simulink model "main"  (R2025b)
settings: Solver=ode1  StartTime=0.0  StopTime=config.sim.var.sim_time  FixedStep=config.sim.var.time_step  RelTol=1e-3
PreLoadFcn:
  | addpath(fullfile(pwd,'images'));
InitFcn:
  | run(fullfile(fileparts(get_param(bdroot,'FileName')),'initializer.mlx'))
StopFcn:
  | run(fullfile(fileparts(get_param(bdroot,'FileName')),'plot/plotting_results.m'))
undefined symbols (not defined in the file): config
libraries: simulink x8, sharedTrackingLibrary x2
(part 1 of 2)
settings Model: Creator=Diogo Lima  LastModifiedBy=Diogo Lima
settings DataIOCC: ExternalInput=config

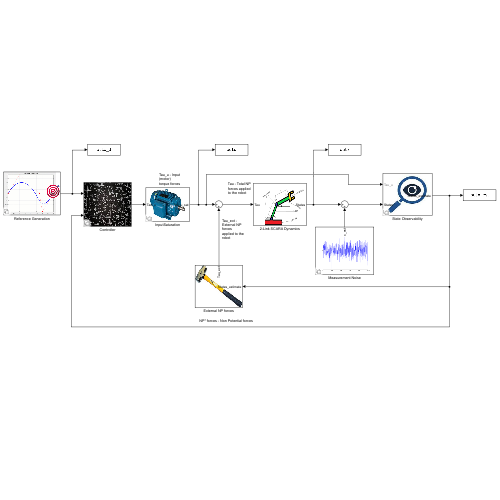
[thumbnail: Simulink's stored preview of the top-level diagram]
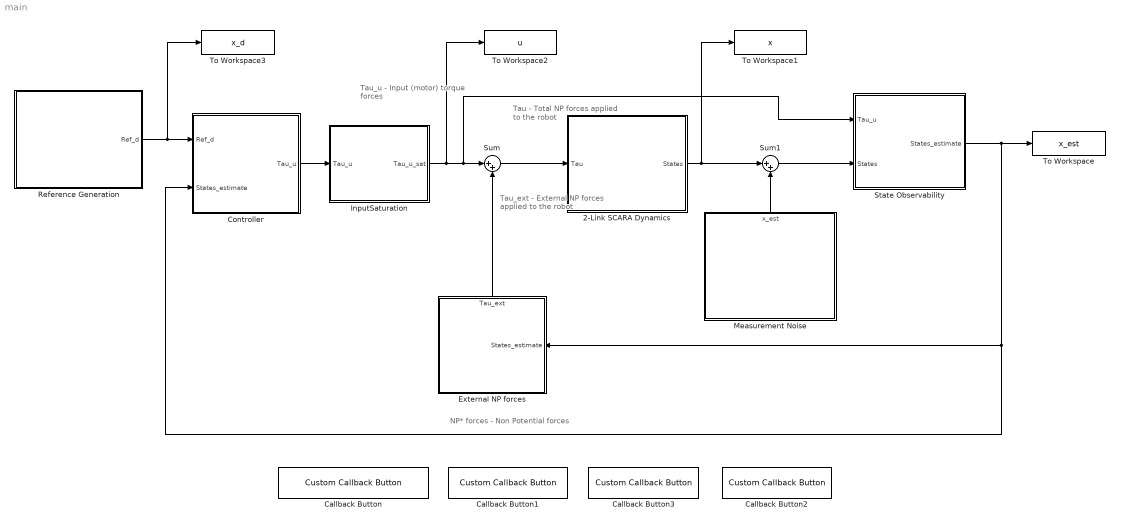
== system main ==
  note: NP* forces - Non Potential forces
  note: Tau - Total NP forces applied to the robot
  note: Tau_u - Input (motor) torque forces
  note: Tau_ext - External NP forces applied to the robot
  2-Link SCARA Dynamics : Subsystem
      mask Display: image('2_Link_Rob_Arm.png');
  Callback Button : CustomCallbackButton  Configuration="{\"components\":[{\"name\":\"BackgroundImageComponent\",\"settings\":{\"image\":{\"size\":[0,0],\"src\":\"default\",\"srcOrientation\":\"Right\"},\"position\":[0,0,1,1]}},{\"name\":\"ButtonStateComponent\",\"settings\":{\"buttonType\":\"momentary\",\"clickFcn\":\"PlotStatesEstDes(plotData);\",\"onValue\":1,\"position\":[0,0,1,1],\"pressDelay\":\"500\",\"pressFcn\":\"\",\"repeatInterval\":\"0\",\"states\":[{\"horizontalAlignment\":\"center\",\"image\":{\"position\":[0,0,1,1],\"size\":[1,1],\"src\":\"default\",\"srcOrientation\":\"Right\"},\"label\":{\"color\":[0.01176470588,0.01176470588,0.01176470588,1],\"icon\":{\"size\":[0,0],\"src\":\"default\",\"srcOrientation\":\"Right\"},\"iconOffset\":0,\"iconPlacement\":\"left\",\"opacity\":1,\"show\":true,\"text\":{\"content\":\"Plot x, x_est and x_d\",\"font\":\"Helvetica\"}},\"labelOffset\":[0,0],\"verticalAlignment\":\"middle\"},{\"horizontalAlignment\":\"center\",\"image\":{\"position\":[0,0,1,1],\"size\":[1,1],\"src\":\"default\",\"srcOrientation\":\"Right\"},\"label\":{\"color\":[0.01176470588,0.01176470588,0.01176470588,1],\"icon\":{\"size\":[0,0],\"src\":\"default\",\"srcOrientation\":\"Right\"},\"iconOffset\":0,\"iconPlacement\":\"left\",\"opacity\":1,\"show\":true,\"text\":{\"content\":\"Plot x, x_est and x_d\",\"font\":\"Helvetica\"}},\"labelOffset\":[0,0],\"verticalAlignment\":\"middle\"},{\"horizontalAlignment\":\"center\",\"image\":{\"position\":[0,0,1,1],\"size\":[1,1],\"src\":\"default\",\"srcOrientation\":\"Right\"},\"label\":{\"color\":[0.01176470588,0.01176470588,0.01176470588,1],\"icon\":{\"size\":[0,0],\"src\":\"default\",\"srcOrientation\":\"Right\"},\"iconOffset\":0,\"iconPlacement\":\"left\",\"opacity\":1,\"show\":true,\"text\":{\"content\":\"Plot x, x_est and x_d\",\"font\":\"Helvetica\"}},\"labelOffset\":[0,0],\"verticalAlignment\":\"middle\"},{\"horizontalAlignment\":\"center\",\"image\":{\"position\":[0,0,1,1],\"size\":[1,1],\"src\":\"default\",\"srcOrientation\":\"Right\"},\"label\":{\"color\":[0.01176470588,0.01176470588,0.01176470588,1],\"icon\":{\"size\":[0,0],\"src\":\"default\",\"srcOrientation\":\"Right\"},\"iconOffset\":0,\"iconPlacement\":\"left\",\"opacity\":1,\"show\":true,\"text\":{\"content\":\"Plot x, x_est and x_d\",\"font\":\"Helvetica\"}},\"labelOffset\":[0,0],\"verticalAlignment\":\"middle\"}]}},{\"name\":\"ForegroundImageComponent\",\"settings\":{\"image\":{\"size\":[0,0],\"src\":\"default\",\"srcOrientation\":\"Right\"},\"isForeground\":1,\"position\":[0,0,1,1]}}],\"derived\":{\"blockParameters\":{\"AutoActivate\":true,\"ButtonText\":\"Plot x, x_est and x_d\",\"ButtonType\":\"Momentary\",\"ClickFcn\":\"PlotStatesEstDes(plotData);\",\"OnValue\":1,\"PressDelay\":\"500\",\"PressFcn\":\"\",\"RepeatInterval\":\"0\",\"fixedAspectRatio\":\"off\"}},\"settings\":{\"BindingType\":\"standalone\",\"autoActivate\":true,\"backgroundColor\":[244,244,244,1],\"backgroundOffset\":0.2,\"backgroundOpacity\":1,\"fixedAspectRatio\":\"off\",\"foregroundColor\":[0.01176470588,0.01176470588,0.01176470588,1],\"migratedFromLegacy\":true,\"useBackgroundColor\":true,\"variant\":\"callback\",\"version\":\"R2025a\"},\"type\":\"Button\"}"  CustomBackgroundColor="{\"color\":[0.9568627451,0.9568627451,0.9568627451],\"show\":true}"
  Callback Button1 : CustomCallbackButton  Configuration="{\"components\":[{\"name\":\"BackgroundImageComponent\",\"settings\":{\"image\":{\"size\":[0,0],\"src\":\"default\",\"srcOrientation\":\"Right\"},\"position\":[0,0,1,1]}},{\"name\":\"ButtonStateComponent\",\"settings\":{\"buttonType\":\"momentary\",\"clickFcn\":\"PlotError(plotData, config);\",\"onValue\":1,\"position\":[0,0,1,1],\"pressDelay\":\"500\",\"pressFcn\":\"\",\"repeatInterval\":\"0\",\"states\":[{\"horizontalAlignment\":\"center\",\"image\":{\"position\":[0,0,1,1],\"size\":[1,1],\"src\":\"default\",\"srcOrientation\":\"Right\"},\"label\":{\"color\":[0.01176470588,0.01176470588,0.01176470588,1],\"icon\":{\"size\":[0,0],\"src\":\"default\",\"srcOrientation\":\"Right\"},\"iconOffset\":0,\"iconPlacement\":\"left\",\"opacity\":1,\"show\":true,\"text\":{\"content\":\"Plot Errors\",\"font\":\"Helvetica\"}},\"labelOffset\":[0,0],\"verticalAlignment\":\"middle\"},{\"horizontalAlignment\":\"center\",\"image\":{\"position\":[0,0,1,1],\"size\":[1,1],\"src\":\"default\",\"srcOrientation\":\"Right\"},\"label\":{\"color\":[0.01176470588,0.01176470588,0.01176470588,1],\"icon\":{\"size\":[0,0],\"src\":\"default\",\"srcOrientation\":\"Right\"},\"iconOffset\":0,\"iconPlacement\":\"left\",\"opacity\":1,\"show\":true,\"text\":{\"content\":\"Plot Errors\",\"font\":\"Helvetica\"}},\"labelOffset\":[0,0],\"verticalAlignment\":\"middle\"},{\"horizontalAlignment\":\"center\",\"image\":{\"position\":[0,0,1,1],\"size\":[1,1],\"src\":\"default\",\"srcOrientation\":\"Right\"},\"label\":{\"color\":[0.01176470588,0.01176470588,0.01176470588,1],\"icon\":{\"size\":[0,0],\"src\":\"default\",\"srcOrientation\":\"Right\"},\"iconOffset\":0,\"iconPlacement\":\"left\",\"opacity\":1,\"show\":true,\"text\":{\"content\":\"Plot Errors\",\"font\":\"Helvetica\"}},\"labelOffset\":[0,0],\"verticalAlignment\":\"middle\"},{\"horizontalAlignment\":\"center\",\"image\":{\"position\":[0,0,1,1],\"size\":[1,1],\"src\":\"default\",\"srcOrientation\":\"Right\"},\"label\":{\"color\":[0.01176470588,0.01176470588,0.01176470588,1],\"icon\":{\"size\":[0,0],\"src\":\"default\",\"srcOrientation\":\"Right\"},\"iconOffset\":0,\"iconPlacement\":\"left\",\"opacity\":1,\"show\":true,\"text\":{\"content\":\"Plot Errors\",\"font\":\"Helvetica\"}},\"labelOffset\":[0,0],\"verticalAlignment\":\"middle\"}]}},{\"name\":\"ForegroundImageComponent\",\"settings\":{\"image\":{\"size\":[0,0],\"src\":\"default\",\"srcOrientation\":\"Right\"},\"isForeground\":1,\"position\":[0,0,1,1]}}],\"derived\":{\"blockParameters\":{\"AutoActivate\":true,\"ButtonText\":\"Plot Errors\",\"ButtonType\":\"Momentary\",\"ClickFcn\":\"PlotError(plotData, config);\",\"OnValue\":1,\"PressDelay\":\"500\",\"PressFcn\":\"\",\"RepeatInterval\":\"0\",\"fixedAspectRatio\":\"off\"}},\"settings\":{\"BindingType\":\"standalone\",\"autoActivate\":true,\"backgroundColor\":[244,244,244,1],\"backgroundOffset\":0.2,\"backgroundOpacity\":1,\"fixedAspectRatio\":\"off\",\"foregroundColor\":[0.01176470588,0.01176470588,0.01176470588,1],\"migratedFromLegacy\":true,\"useBackgroundColor\":true,\"variant\":\"callback\",\"version\":\"R2025a\"},\"type\":\"Button\"}"  CustomBackgroundColor="{\"color\":[0.9568627451,0.9568627451,0.9568627451],\"show\":true}"
  Callback Button2 : CustomCallbackButton  Configuration="{\"components\":[{\"name\":\"BackgroundImageComponent\",\"settings\":{\"image\":{\"size\":[0,0],\"src\":\"default\",\"srcOrientation\":\"Right\"},\"position\":[0,0,1,1]}},{\"name\":\"ButtonStateComponent\",\"settings\":{\"buttonType\":\"momentary\",\"clickFcn\":\"Animate2LinkSCARA(plotData, config);\",\"onValue\":1,\"position\":[0,0,1,1],\"pressDelay\":\"500\",\"pressFcn\":\"\",\"repeatInterval\":\"0\",\"states\":[{\"horizontalAlignment\":\"center\",\"image\":{\"position\":[0,0,1,1],\"size\":[1,1],\"src\":\"default\",\"srcOrientation\":\"Right\"},\"label\":{\"color\":[0.01176470588,0.01176470588,0.01176470588,1],\"icon\":{\"size\":[0,0],\"src\":\"default\",\"srcOrientation\":\"Right\"},\"iconOffset\":0,\"iconPlacement\":\"left\",\"opacity\":1,\"show\":true,\"text\":{\"content\":\"Animation\",\"font\":\"Helvetica\"}},\"labelOffset\":[0,0],\"verticalAlignment\":\"middle\"},{\"horizontalAlignment\":\"center\",\"image\":{\"position\":[0,0,1,1],\"size\":[1,1],\"src\":\"default\",\"srcOrientation\":\"Right\"},\"label\":{\"color\":[0.01176470588,0.01176470588,0.01176470588,1],\"icon\":{\"size\":[0,0],\"src\":\"default\",\"srcOrientation\":\"Right\"},\"iconOffset\":0,\"iconPlacement\":\"left\",\"opacity\":1,\"show\":true,\"text\":{\"content\":\"Animation\",\"font\":\"Helvetica\"}},\"labelOffset\":[0,0],\"verticalAlignment\":\"middle\"},{\"horizontalAlignment\":\"center\",\"image\":{\"position\":[0,0,1,1],\"size\":[1,1],\"src\":\"default\",\"srcOrientation\":\"Right\"},\"label\":{\"color\":[0.01176470588,0.01176470588,0.01176470588,1],\"icon\":{\"size\":[0,0],\"src\":\"default\",\"srcOrientation\":\"Right\"},\"iconOffset\":0,\"iconPlacement\":\"left\",\"opacity\":1,\"show\":true,\"text\":{\"content\":\"Animation\",\"font\":\"Helvetica\"}},\"labelOffset\":[0,0],\"verticalAlignment\":\"middle\"},{\"horizontalAlignment\":\"center\",\"image\":{\"position\":[0,0,1,1],\"size\":[1,1],\"src\":\"default\",\"srcOrientation\":\"Right\"},\"label\":{\"color\":[0.01176470588,0.01176470588,0.01176470588,1],\"icon\":{\"size\":[0,0],\"src\":\"default\",\"srcOrientation\":\"Right\"},\"iconOffset\":0,\"iconPlacement\":\"left\",\"opacity\":1,\"show\":true,\"text\":{\"content\":\"Animation\",\"font\":\"Helvetica\"}},\"labelOffset\":[0,0],\"verticalAlignment\":\"middle\"}]}},{\"name\":\"ForegroundImageComponent\",\"settings\":{\"image\":{\"size\":[0,0],\"src\":\"default\",\"srcOrientation\":\"Right\"},\"isForeground\":1,\"position\":[0,0,1,1]}}],\"derived\":{\"blockParameters\":{\"AutoActivate\":true,\"ButtonText\":\"Animation\",\"ButtonType\":\"Momentary\",\"ClickFcn\":\"Animate2LinkSCARA(plotData, config);\",\"OnValue\":1,\"PressDelay\":\"500\",\"PressFcn\":\"\",\"RepeatInterval\":\"0\",\"fixedAspectRatio\":\"off\"}},\"settings\":{\"BindingType\":\"standalone\",\"autoActivate\":true,\"backgroundColor\":[244,244,244,1],\"backgroundOffset\":0.2,\"backgroundOpacity\":1,\"fixedAspectRatio\":\"off\",\"foregroundColor\":[0.01176470588,0.01176470588,0.01176470588,1],\"migratedFromLegacy\":true,\"useBackgroundColor\":true,\"variant\":\"callback\",\"version\":\"R2025a\"},\"type\":\"Button\"}"  CustomBackgroundColor="{\"color\":[0.9568627451,0.9568627451,0.9568627451],\"show\":true}"
  Callback Button3 : CustomCallbackButton  Configuration="{\"components\":[{\"name\":\"BackgroundImageComponent\",\"settings\":{\"image\":{\"size\":[0,0],\"src\":\"default\",\"srcOrientation\":\"Right\"},\"position\":[0,0,1,1]}},{\"name\":\"ButtonStateComponent\",\"settings\":{\"buttonType\":\"momentary\",\"clickFcn\":\"PlotInput(plotData, config);\",\"onValue\":1,\"position\":[0,0,1,1],\"pressDelay\":\"500\",\"pressFcn\":\"\",\"repeatInterval\":\"0\",\"states\":[{\"horizontalAlignment\":\"center\",\"image\":{\"position\":[0,0,1,1],\"size\":[1,1],\"src\":\"default\",\"srcOrientation\":\"Right\"},\"label\":{\"color\":[0.01176470588,0.01176470588,0.01176470588,1],\"icon\":{\"size\":[0,0],\"src\":\"default\",\"srcOrientation\":\"Right\"},\"iconOffset\":0,\"iconPlacement\":\"left\",\"opacity\":1,\"show\":true,\"text\":{\"content\":\"Input Torques\",\"font\":\"Helvetica\"}},\"labelOffset\":[0,0],\"verticalAlignment\":\"middle\"},{\"horizontalAlignment\":\"center\",\"image\":{\"position\":[0,0,1,1],\"size\":[1,1],\"src\":\"default\",\"srcOrientation\":\"Right\"},\"label\":{\"color\":[0.01176470588,0.01176470588,0.01176470588,1],\"icon\":{\"size\":[0,0],\"src\":\"default\",\"srcOrientation\":\"Right\"},\"iconOffset\":0,\"iconPlacement\":\"left\",\"opacity\":1,\"show\":true,\"text\":{\"content\":\"Input Torques\",\"font\":\"Helvetica\"}},\"labelOffset\":[0,0],\"verticalAlignment\":\"middle\"},{\"horizontalAlignment\":\"center\",\"image\":{\"position\":[0,0,1,1],\"size\":[1,1],\"src\":\"default\",\"srcOrientation\":\"Right\"},\"label\":{\"color\":[0.01176470588,0.01176470588,0.01176470588,1],\"icon\":{\"size\":[0,0],\"src\":\"default\",\"srcOrientation\":\"Right\"},\"iconOffset\":0,\"iconPlacement\":\"left\",\"opacity\":1,\"show\":true,\"text\":{\"content\":\"Input Torques\",\"font\":\"Helvetica\"}},\"labelOffset\":[0,0],\"verticalAlignment\":\"middle\"},{\"horizontalAlignment\":\"center\",\"image\":{\"position\":[0,0,1,1],\"size\":[1,1],\"src\":\"default\",\"srcOrientation\":\"Right\"},\"label\":{\"color\":[0.01176470588,0.01176470588,0.01176470588,1],\"icon\":{\"size\":[0,0],\"src\":\"default\",\"srcOrientation\":\"Right\"},\"iconOffset\":0,\"iconPlacement\":\"left\",\"opacity\":1,\"show\":true,\"text\":{\"content\":\"Input Torques\",\"font\":\"Helvetica\"}},\"labelOffset\":[0,0],\"verticalAlignment\":\"middle\"}]}},{\"name\":\"ForegroundImageComponent\",\"settings\":{\"image\":{\"size\":[0,0],\"src\":\"default\",\"srcOrientation\":\"Right\"},\"isForeground\":1,\"position\":[0,0,1,1]}}],\"derived\":{\"blockParameters\":{\"AutoActivate\":true,\"ButtonText\":\"Input Torques\",\"ButtonType\":\"Momentary\",\"ClickFcn\":\"PlotInput(plotData, config);\",\"OnValue\":1,\"PressDelay\":\"500\",\"PressFcn\":\"\",\"RepeatInterval\":\"0\",\"fixedAspectRatio\":\"off\"}},\"settings\":{\"BindingType\":\"standalone\",\"autoActivate\":true,\"backgroundColor\":[244,244,244,1],\"backgroundOffset\":0.2,\"backgroundOpacity\":1,\"fixedAspectRatio\":\"off\",\"foregroundColor\":[0.01176470588,0.01176470588,0.01176470588,1],\"migratedFromLegacy\":true,\"useBackgroundColor\":true,\"variant\":\"callback\",\"version\":\"R2025a\"},\"type\":\"Button\"}"  CustomBackgroundColor="{\"color\":[0.9568627451,0.9568627451,0.9568627451],\"show\":true}"
  Controller : Subsystem  Variant=on  VariantActivationTime=inherit from Simulink.VariantControl
      mask Display: image('math.jpeg');
  External NP forces : Subsystem
      settings: PortSchema="{\"entries\":[{\"content\":{\"sides\":[{\"content\":{},\"type\":\"ConnectorPlacement.EquallySpacedRectSide\",\"uuid\":\"ab8935ab-44b5-4f89-9c76-b9cab063ccb6\"},{\"content\":{\"connectorIds\":[\"In1\"],\"side\":\"RIGHT\"},\"type\":\"ConnectorPlacement.EquallySpacedRectSide\",\"uuid\":\"7b95b46e-af84-4841-baf6-a25fb8fbec5d\"},{\"content\":{\"connectorIds\":[\"Out1\"],\"side\":\"TOP\"},\"type\":\"ConnectorPlacement.EquallySpacedRectSide\",\"uuid\":\"f47b6b94-5272-4357-86f1-013d8bd46a68\"},{\"content\":{\"side\":\"BOTTOM\"},\"type\":\"ConnectorPlacement.EquallySpacedRectSide\",\"uuid\":\"e5ddd4d5-8d82-42eb-baf0-e1f1d67c3ee6\"}]},\"type\":\"ConnectorPlacement.EquallySpacedConnector\",\"uuid\":\"5043c8e4-624e-44a2-8db2-4a7bf2c36b25\"}],\"packageUris\":[\"http://schema.mathworks.com/mf0/Connector/R2020b\"],\"version\":\"1.0\"}"
      mask Display: image('hammer.jpeg');
  InputSaturation : Subsystem  Variant=on  VariantActivationTime=inherit from Simulink.VariantControl
      mask Display: image('eetric motor.jpeg');
  Measurement Noise : Subsystem  Variant=on  VariantActivationTime=inherit from Simulink.VariantControl
      settings: PortSchema="{\"entries\":[{\"content\":{\"sides\":[{\"content\":{},\"type\":\"ConnectorPlacement.EquallySpacedRectSide\",\"uuid\":\"d15af3bb-429c-4511-867e-2dbe032e8cba\"},{\"content\":{\"side\":\"RIGHT\"},\"type\":\"ConnectorPlacement.EquallySpacedRectSide\",\"uuid\":\"fe1fb238-6986-44a7-806c-ef391cb9083b\"},{\"content\":{\"connectorIds\":[\"Out1\"],\"side\":\"TOP\"},\"type\":\"ConnectorPlacement.EquallySpacedRectSide\",\"uuid\":\"1cb65108-e0a3-4597-9e58-247715da98e5\"}]},\"type\":\"ConnectorPlacement.EquallySpacedConnector\",\"uuid\":\"dec8af6e-1fcd-4cfd-bd39-6a634de96718\"}],\"packageUris\":[\"http://schema.mathworks.com/mf0/Connector/R2020b\"],\"version\":\"1.0\"}"
      mask Display: image('gussian_normal_noise.png');
  Reference Generation : Subsystem  Variant=on  VariantActivationTime=inherit from Simulink.VariantControl
      mask Display: image('Trajectory Target.png');
  State Observability : Subsystem  Variant=on  VariantActivationTime=inherit from Simulink.VariantControl
      mask Display: image('magnifying glass.jpeg');
  Sum : Sum  Inputs=|++
  Sum1 : Sum  Inputs=|++
  To Workspace : ToWorkspace  VariableName=x_est  SaveFormat=Structure With Time  SampleTime=-1
  To Workspace1 : ToWorkspace  VariableName=x  SaveFormat=Structure With Time  SampleTime=-1
  To Workspace2 : ToWorkspace  VariableName=u  SaveFormat=Structure With Time  SampleTime=-1
  To Workspace3 : ToWorkspace  VariableName=x_d  SaveFormat=Structure With Time  SampleTime=-1
  wires:
  2-Link SCARA Dynamics/1(States) -> Sum1/1, To Workspace1/1
  Sum/1 -> 2-Link SCARA Dynamics/1(Tau)
  External NP forces/1(Tau_ext) -> Sum/2
  Reference Generation/1(Ref_d) -> To Workspace3/1, Controller/1(Ref_d)
  Controller/1(Tau_u) -> InputSaturation/1(Tau_u)
  InputSaturation/1(Tau_u_sat) -> To Workspace2/1, State Observability/1(Tau_u), Sum/1
  State Observability/1(States_estimate) -> Controller/2(States_estimate), External NP forces/1(States_estimate), To Workspace/1
  Sum1/1 -> State Observability/2(States)
  Measurement Noise/1(x_est) -> Sum1/2

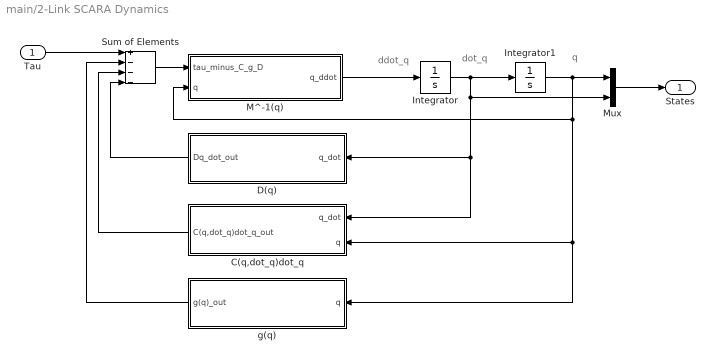
== system main/2-Link SCARA Dynamics ==
  note: dot_q
  note: q
  note: ddot_q
  Tau : Inport
  C(q,dot_q)dot_q : Subsystem
      settings: PortSchema="{\"entries\":[{\"content\":{\"sides\":[{\"content\":{\"connectorIds\":[\"Out1\"]},\"type\":\"ConnectorPlacement.EquallySpacedRectSide\",\"uuid\":\"e2ae5650-0784-458d-831f-709044d8d2e7\"},{\"content\":{\"connectorIds\":[\"In1\",\"In2\"],\"side\":\"RIGHT\"},\"type\":\"ConnectorPlacement.EquallySpacedRectSide\",\"uuid\":\"7d6ada7b-e0cb-4ab5-ae4d-653c8188ff73\"},{\"content\":{\"side\":\"TOP\"},\"type\":\"ConnectorPlacement.EquallySpacedRectSide\",\"uuid\":\"6bba282a-332d-41c7-9399-ff8c7d6086e4\"}]},\"type\":\"ConnectorPlacement.EquallySpacedConnector\",\"uuid\":\"9d2ac4ef-2b70-4a02-8c87-fdaaf2184e3a\"}],\"packageUris\":[\"http://schema.mathworks.com/mf0/Connector/R2020b\"],\"version\":\"1.0\"}"
  D(q) : Subsystem
      settings: PortSchema="{\"entries\":[{\"content\":{\"sides\":[{\"content\":{\"connectorIds\":[\"Out1\"]},\"type\":\"ConnectorPlacement.EquallySpacedRectSide\",\"uuid\":\"e2ae5650-0784-458d-831f-709044d8d2e7\"},{\"content\":{\"connectorIds\":[\"In1\"],\"side\":\"RIGHT\"},\"type\":\"ConnectorPlacement.EquallySpacedRectSide\",\"uuid\":\"7d6ada7b-e0cb-4ab5-ae4d-653c8188ff73\"},{\"content\":{\"side\":\"TOP\"},\"type\":\"ConnectorPlacement.EquallySpacedRectSide\",\"uuid\":\"6bba282a-332d-41c7-9399-ff8c7d6086e4\"}]},\"type\":\"ConnectorPlacement.EquallySpacedConnector\",\"uuid\":\"9d2ac4ef-2b70-4a02-8c87-fdaaf2184e3a\"}],\"packageUris\":[\"http://schema.mathworks.com/mf0/Connector/R2020b\"],\"version\":\"1.0\"}"
  Integrator : Integrator  InitialCondition=config.sim.var.init_cond.ang_vel
  Integrator1 : Integrator  InitialCondition=config.sim.var.init_cond.ang_pos
  M^-1(q) : Subsystem
  Mux : Mux  Inputs=2
  Sum of Elements : Sum  Inputs=+---
  g(q) : Subsystem
      settings: PortSchema="{\"entries\":[{\"content\":{\"sides\":[{\"content\":{\"connectorIds\":[\"Out1\"]},\"type\":\"ConnectorPlacement.EquallySpacedRectSide\",\"uuid\":\"e2ae5650-0784-458d-831f-709044d8d2e7\"},{\"content\":{\"connectorIds\":[\"In1\"],\"side\":\"RIGHT\"},\"type\":\"ConnectorPlacement.EquallySpacedRectSide\",\"uuid\":\"7d6ada7b-e0cb-4ab5-ae4d-653c8188ff73\"},{\"content\":{\"side\":\"TOP\"},\"type\":\"ConnectorPlacement.EquallySpacedRectSide\",\"uuid\":\"6bba282a-332d-41c7-9399-ff8c7d6086e4\"}]},\"type\":\"ConnectorPlacement.EquallySpacedConnector\",\"uuid\":\"9d2ac4ef-2b70-4a02-8c87-fdaaf2184e3a\"}],\"packageUris\":[\"http://schema.mathworks.com/mf0/Connector/R2020b\"],\"version\":\"1.0\"}"
  States : Outport
  wires:
  M^-1(q)/1(q_ddot) -> Integrator/1
  Integrator/1 -> C(q,dot_q)dot_q/1(q_dot), D(q)/1(q_dot), Mux/2, Integrator1/1
  Mux/1 -> States/1
  Integrator1/1 -> M^-1(q)/2(q), g(q)/1(q), C(q,dot_q)dot_q/2(q), Mux/1
  Sum of Elements/1 -> M^-1(q)/1(tau_minus_C_g_D)
  Tau/1 -> Sum of Elements/1
  D(q)/1(Dq_dot_out) -> Sum of Elements/4
  C(q,dot_q)dot_q/1(C(q,dot_q)dot_q_out) -> Sum of Elements/3
  g(q)/1(g(q)_out) -> Sum of Elements/2

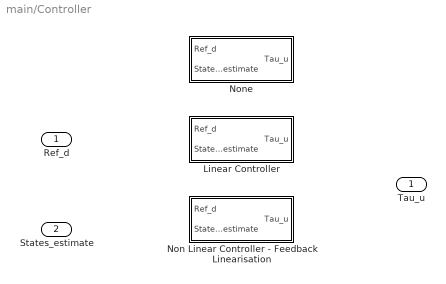
== system main/Controller ==
  Ref_d : Inport
  States_estimate : Inport  Port=2
  Linear Controller : Subsystem  VariantControl=ControllerSel == ControllerType.LinearSS
  Non Linear Controller - Feedback Linearisation : Subsystem  VariantControl=ControllerSel == ControllerType.NonLinearFL
  None : Subsystem  VariantControl=ControllerSel == ControllerType.None
  Tau_u : Outport

== system main/External NP forces ==
  States_estimate : Inport
  Add : Sum
  External Disturbance Forces / Model Uncertainties : Subsystem  Variant=on  VariantActivationTime=inherit from Simulink.VariantControl
      mask Display: image('wind.png');
  Payload : Subsystem  Variant=on  VariantActivationTime=inherit from Simulink.VariantControl
      mask Display: image('coca_cola_can.jpeg');
  Tau_ext : Outport
  wires:
  States_estimate/1 -> Payload/1(States_estimate)
  Payload/1(Tau_payload) -> Add/1
  Add/1 -> Tau_ext/1
  External Disturbance Forces / Model Uncertainties/1(Tau_ext) -> Add/2

== system main/InputSaturation ==
  Tau_u : Inport
  Active : Subsystem  VariantControl=InputSaturationSel == InputSaturation.Active
  Not Active : Subsystem  VariantControl=InputSaturationSel == InputSaturation.NotActive
  Tau_u_sat : Outport

== system main/Measurement Noise ==
  Gaussian Noise : Subsystem  VariantControl=MeasDisturbancesSel == MeasDisturbances.GaussianDisturbance
  None : Subsystem  VariantControl=MeasDisturbancesSel == MeasDisturbances.None
  x_est : Outport

== system main/Reference Generation ==
  Regulation : Subsystem  VariantControl=RefGenerationSel == RefGeneration.Regulation
  Trajectory : Subsystem  VariantControl=RefGenerationSel == RefGeneration.Trajectory
  Ref_d : Outport

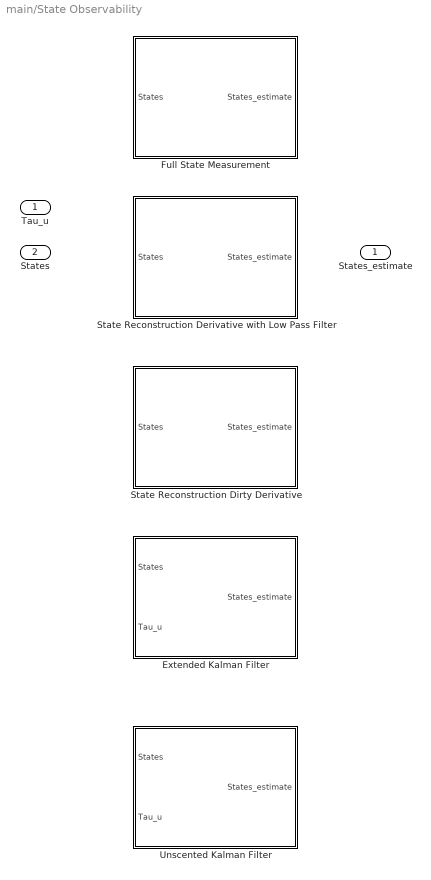
== system main/State Observability ==
  Tau_u : Inport
  States : Inport  Port=2
  Extended Kalman Filter : Subsystem  VariantControl=StateObservabilitySel == StateObservability.ExtendedKalmanBucyFilter
  Full State Measurement : Subsystem  VariantControl=StateObservabilitySel == StateObservability.FullStateMeasurement
  State Reconstruction Derivative with Low Pass Filter : Subsystem  VariantControl=StateObservabilitySel == StateObservability.StateReconstructionDevLowPassFilt
  State Reconstruction Dirty Derivative : Subsystem  VariantControl=StateObservabilitySel == StateObservability.StateReconstructionDirtyDev
  Unscented Kalman Filter : Subsystem  VariantControl=StateObservabilitySel == StateObservability.UnscentedKalmanFilter
  States_estimate : Outport

== system main/2-Link SCARA Dynamics/C(q,dot_q)dot_q ==
  q_dot : Inport
  q : Inport  Port=2
  C(q,dot_q)dot_q : MATLAB Function  TreatAsAtomicUnit=on
  C(q,dot_q)dot_q_out : Outport
  wires:
  q_dot/1 -> C(q,dot_q)dot_q/2(q_dot)
  C(q,dot_q)dot_q/1(output) -> C(q,dot_q)dot_q_out/1
  q/1 -> C(q,dot_q)dot_q/1(q)

== system main/2-Link SCARA Dynamics/D(q) ==
  q_dot : Inport
  Dq_dot : MATLAB Function  TreatAsAtomicUnit=on
  Dq_dot_out : Outport
  wires:
  q_dot/1 -> Dq_dot/1(q_dot)
  Dq_dot/1(output) -> Dq_dot_out/1

== system main/2-Link SCARA Dynamics/M^-1(q) ==
  tau_minus_C_g_D : Inport
  q : Inport  Port=2
  M^-1(q) : MATLAB Function  TreatAsAtomicUnit=on
  q_ddot : Outport
  wires:
  M^-1(q)/1(output) -> q_ddot/1
  tau_minus_C_g_D/1 -> M^-1(q)/2(tau_minus_C_g_D)
  q/1 -> M^-1(q)/1(q)

== system main/2-Link SCARA Dynamics/g(q) ==
  q : Inport
  g(q) : MATLAB Function  TreatAsAtomicUnit=on
  g(q)_out : Outport
  wires:
  q/1 -> g(q)/1(q)
  g(q)/1(output) -> g(q)_out/1

== system main/Controller/Linear Controller ==
  Ref_d : Inport
  States_estimate : Inport  Port=2
  Tau_u : Outport

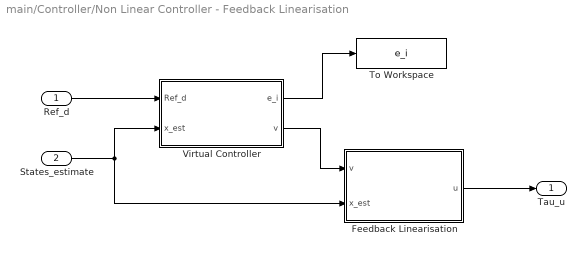
== system main/Controller/Non Linear Controller - Feedback Linearisation ==
  Ref_d : Inport
  States_estimate : Inport  Port=2
  Feedback Linearisation : MATLAB Function  TreatAsAtomicUnit=on
  To Workspace : ToWorkspace  VariableName=e_i  SaveFormat=Structure With Time  SampleTime=-1
  Virtual Controller : MATLAB Function  TreatAsAtomicUnit=on
  Tau_u : Outport
  wires:
  States_estimate/1 -> Virtual Controller/2(x_est), Feedback Linearisation/2(x_est)
  Ref_d/1 -> Virtual Controller/1(Ref_d)
  Virtual Controller/2(v) -> Feedback Linearisation/1(v)
  Feedback Linearisation/1(u) -> Tau_u/1
  Virtual Controller/1(e_i) -> To Workspace/1

== system main/Controller/None ==
  Ref_d : Inport
  States_estimate : Inport  Port=2
  Constant : Constant  Value=[0;0]
  Tau_u : Outport
  wires:
  Constant/1 -> Tau_u/1

== system main/External NP forces/External Disturbance Forces // Model Uncertainties ==
  Constant Force : Subsystem  VariantControl=ExtDisturbancesSel == ExtDisturbances.ConstForce
  Gaussian Force : Subsystem  VariantControl=ExtDisturbancesSel == ExtDisturbances.GaussianForce
  Gaussian and Constant Force : Subsystem  VariantControl=ExtDisturbancesSel == ExtDisturbances.GaussianAndConstForce
  None : Subsystem  VariantControl=ExtDisturbancesSel == ExtDisturbances.None
  Tau_ext : Outport

== system main/External NP forces/Payload ==
  States_estimate : Inport
  None : Subsystem  VariantControl=PayloadSel == Payload.None
  Payload : Subsystem  VariantControl=PayloadSel == Payload.Constant
  Tau_payload : Outport

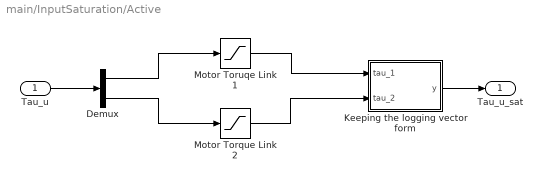
== system main/InputSaturation/Active ==
  Tau_u : Inport
  Demux : Demux  Outputs=2
  Keeping the logging vector form : MATLAB Function  TreatAsAtomicUnit=on
  Motor Torque Link 2 : Saturate  UpperLimit=config.robot.motor.saturation.joint_2  LowerLimit=-config.robot.motor.saturation.joint_2
  Motor Toruqe Link 1 : Saturate  UpperLimit=config.robot.motor.saturation.joint_1  LowerLimit=-config.robot.motor.saturation.joint_1
  Tau_u_sat : Outport
  wires:
  Tau_u/1 -> Demux/1
  Demux/1 -> Motor Toruqe Link 1/1
  Demux/2 -> Motor Torque Link 2/1
  Motor Toruqe Link 1/1 -> Keeping the logging vector form/1(tau_1)
  Motor Torque Link 2/1 -> Keeping the logging vector form/2(tau_2)
  Keeping the logging vector form/1(y) -> Tau_u_sat/1

== system main/InputSaturation/Not Active ==
  Tau_u : Inport
  Tau_u_sat : Outport
  wires:
  Tau_u/1 -> Tau_u_sat/1

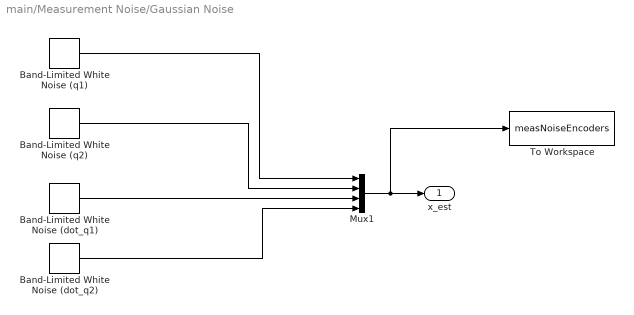
== system main/Measurement Noise/Gaussian Noise ==
  Band-Limited White Noise (dot_q1) : simulink/Sources/Band-Limited White Noise  Cov=config.disturbances.measurements.noise.ang_vel_1.power  Ts=config.disturbances.measurements.noise.encoders.timeStep  seed=[23343]
  Band-Limited White Noise (dot_q2) : simulink/Sources/Band-Limited White Noise  Cov=config.disturbances.measurements.noise.ang_vel_2.power  Ts=config.disturbances.measurements.noise.encoders.timeStep  seed=[23344]
  Band-Limited White Noise (q1) : simulink/Sources/Band-Limited White Noise  Cov=config.disturbances.measurements.noise.encoder_1.power  Ts=config.disturbances.measurements.noise.encoders.timeStep  seed=[23341]
  Band-Limited White Noise (q2) : simulink/Sources/Band-Limited White Noise  Cov=config.disturbances.measurements.noise.encoder_2.power  Ts=config.disturbances.measurements.noise.encoders.timeStep  seed=[23342]
  Mux1 : Mux
  To Workspace : ToWorkspace  VariableName=measNoiseEncoders  SaveFormat=Structure With Time  SampleTime=-1
  x_est : Outport
  wires:
  Mux1/1 -> To Workspace/1, x_est/1
  Band-Limited White Noise (dot_q1)/1 -> Mux1/3
  Band-Limited White Noise (dot_q2)/1 -> Mux1/4
  Band-Limited White Noise (q2)/1 -> Mux1/2
  Band-Limited White Noise (q1)/1 -> Mux1/1

== system main/Measurement Noise/None ==
  Constant : Constant  Value=[0; 0; 0; 0]
  x_est : Outport
  wires:
  Constant/1 -> x_est/1

== system main/Reference Generation/Regulation ==
  Constant : Constant  Value=config.refGeneration.regulation.pos_d
  Ref_d : Outport
  wires:
  Constant/1 -> Ref_d/1

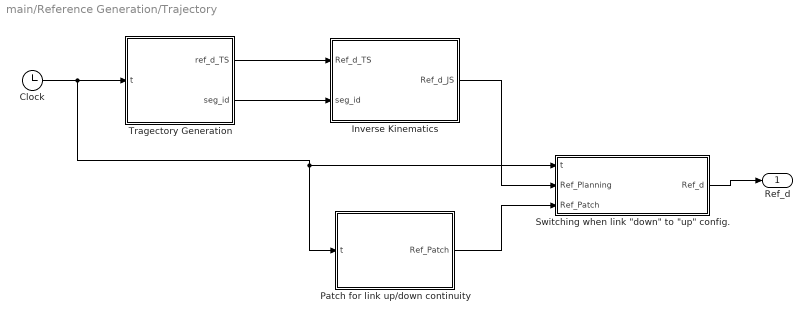
== system main/Reference Generation/Trajectory ==
  Clock : Clock
  Inverse Kinematics : MATLAB Function  TreatAsAtomicUnit=on
  Patch for link up/down continuity : MATLAB Function  TreatAsAtomicUnit=on
  "Switching when link \"down\" to \"up\" config." : MATLAB Function  TreatAsAtomicUnit=on
  Tragectory Generation : MATLAB Function  TreatAsAtomicUnit=on
  Ref_d : Outport
  wires:
  Tragectory Generation/1(ref_d_TS) -> Inverse Kinematics/1(Ref_d_TS)
  Clock/1 -> Patch for link up/down continuity/1(t), "Switching when link \"down\" to \"up\" config."/1(t), Tragectory Generation/1(t)
  Tragectory Generation/2(seg_id) -> Inverse Kinematics/2(seg_id)
  Inverse Kinematics/1(Ref_d_JS) -> "Switching when link \"down\" to \"up\" config."/2(Ref_Planning)
  "Switching when link \"down\" to \"up\" config."/1(Ref_d) -> Ref_d/1
  Patch for link up/down continuity/1(Ref_Patch) -> "Switching when link \"down\" to \"up\" config."/3(Ref_Patch)

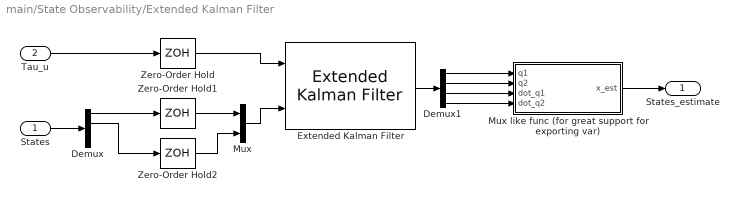
== system main/State Observability/Extended Kalman Filter ==
  States : Inport
  Tau_u : Inport  Port=2
  Demux : Demux
  Demux1 : Demux
  Extended Kalman Filter : sharedTrackingLibrary/Extended Kalman Filter  StateTransitionFcn=myStateTransitionFcn  HasStateTransitionJacobianFcn=on  StateTransitionJacobianFcn=myStateTransitionJacobianFcn  HasAdditiveProcessNoise=Additive  ProcessNoise=config.stateObservability.extKalFil.process_noise  HasTimeVaryingProcessNoise=off  HasStateTransitionFcnExtraArgument=1  InitialState=config.sim.var.init_cond.states_vec  InitialStateCovariance=config.stateObservability.extKalFil.init_state_cov  MeasurementFcn1=myMeasurementFcn  HasMeasurementJacobianFcn1=on  MeasurementJacobianFcn1=myMeasurementJacobianFcn  HasMeasurementEnablePort1=off  HasAdditiveMeasurementNoise1=Additive  MeasurementNoise1=config.stateObservability.extKalFil.meas_noise  HasTimeVaryingMeasurementNoise1=off  HasMeasurementFcnExtraArgument1=0  HasMeasurementWrapping1=off  MeasurementFcn2=myMeasurementFcn  HasMeasurementJacobianFcn2=off  HasMeasurementEnablePort2=off  HasAdditiveMeasurementNoise2=Additive  MeasurementNoise2=1  HasTimeVaryingMeasurementNoise2=off  HasMeasurementFcnExtraArgument2=0  HasMeasurementWrapping2=off  MeasurementFcn3=myMeasurementFcn  HasMeasurementJacobianFcn3=off  HasMeasurementEnablePort3=off  HasAdditiveMeasurementNoise3=Additive  MeasurementNoise3=1  HasTimeVaryingMeasurementNoise3=off  HasMeasurementFcnExtraArgument3=0  HasMeasurementWrapping3=off  MeasurementFcn4=myMeasurementFcn  HasMeasurementJacobianFcn4=off  HasMeasurementEnablePort4=off  HasAdditiveMeasurementNoise4=Additive  MeasurementNoise4=1  HasTimeVaryingMeasurementNoise4=off  HasMeasurementFcnExtraArgument4=0  HasMeasurementWrapping4=off  MeasurementFcn5=myMeasurementFcn  HasMeasurementJacobianFcn5=off  HasMeasurementEnablePort5=off  HasAdditiveMeasurementNoise5=Additive  MeasurementNoise5=1  HasTimeVaryingMeasurementNoise5=off  HasMeasurementFcnExtraArgument5=0  HasMeasurementWrapping5=off  EnableMultirate=off  StateTransitionFcnSampleTime=1  MeasurementFcn1SampleTime=1  MeasurementFcn2SampleTime=1  MeasurementFcn3SampleTime=1  MeasurementFcn4SampleTime=1  MeasurementFcn5SampleTime=1  UseCurrentEstimator=on  OutputStateCovariance=off  DataType=double  SampleTime=config.sim.var.time_step  NumberOfMeasurements=1
  Mux : Mux  Inputs=2
  Mux like func (for great support for exporting var) : MATLAB Function  TreatAsAtomicUnit=on
  Zero-Order Hold : ZeroOrderHold  SampleTime=config.sim.var.time_step
  Zero-Order Hold1 : ZeroOrderHold  SampleTime=config.sim.var.time_step
  Zero-Order Hold2 : ZeroOrderHold  SampleTime=config.sim.var.time_step
  States_estimate : Outport
  wires:
  Tau_u/1 -> Zero-Order Hold/1
  Zero-Order Hold/1 -> Extended Kalman Filter/1
  States/1 -> Demux/1
  Demux/1 -> Zero-Order Hold1/1
  Demux/2 -> Zero-Order Hold2/1
  Mux/1 -> Extended Kalman Filter/2
  Zero-Order Hold1/1 -> Mux/1
  Zero-Order Hold2/1 -> Mux/2
  Mux like func (for great support for exporting var)/1(x_est) -> States_estimate/1
  Extended Kalman Filter/1 -> Demux1/1
  Demux1/1 -> Mux like func (for great support for exporting var)/1(q1)
  Demux1/2 -> Mux like func (for great support for exporting var)/2(q2)
  Demux1/3 -> Mux like func (for great support for exporting var)/3(dot_q1)
  Demux1/4 -> Mux like func (for great support for exporting var)/4(dot_q2)

== system main/State Observability/Full State Measurement ==
  States : Inport
  States_estimate : Outport
  wires:
  States/1 -> States_estimate/1

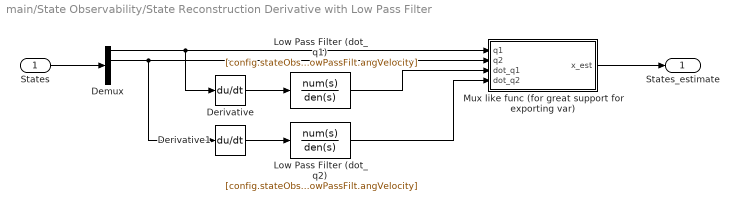
== system main/State Observability/State Reconstruction Derivative with Low Pass Filter ==
  States : Inport
  Demux : Demux
  Derivative : Derivative
  Derivative1 : Derivative
  Low Pass Filter (dot_q1) : TransferFcn  Numerator=[config.stateObservability.stateReconstruction.DevLowPassFilt.angVelocity]  Denominator=[1 config.stateObservability.stateReconstruction.DevLowPassFilt.angVelocity]
  Low Pass Filter (dot_q2) : TransferFcn  Numerator=[config.stateObservability.stateReconstruction.DevLowPassFilt.angVelocity]  Denominator=[1 config.stateObservability.stateReconstruction.DevLowPassFilt.angVelocity]
  Mux like func (for great support for exporting var) : MATLAB Function  TreatAsAtomicUnit=on
  States_estimate : Outport
  wires:
  States/1 -> Demux/1
  Mux like func (for great support for exporting var)/1(x_est) -> States_estimate/1
  Demux/1 -> Mux like func (for great support for exporting var)/1(q1), Derivative/1
  Demux/2 -> Mux like func (for great support for exporting var)/2(q2), Derivative1/1
  Derivative1/1 -> Low Pass Filter (dot_q2)/1
  Derivative/1 -> Low Pass Filter (dot_q1)/1
  Low Pass Filter (dot_q2)/1 -> Mux like func (for great support for exporting var)/4(dot_q2)
  Low Pass Filter (dot_q1)/1 -> Mux like func (for great support for exporting var)/3(dot_q1)

== system main/State Observability/State Reconstruction Dirty Derivative ==
  States : Inport
  Demux : Demux
  Mux like func (for great support for exporting var) : MATLAB Function  TreatAsAtomicUnit=on
  Transfer Fcn : TransferFcn  Numerator=[1 0]  Denominator=[config.stateObservability.stateReconstruction.DirtyDev.timeConst 1]
  Transfer Fcn2 : TransferFcn  Numerator=[1 0]  Denominator=[config.stateObservability.stateReconstruction.DirtyDev.timeConst 1]
  States_estimate : Outport
  wires:
  States/1 -> Demux/1
  Mux like func (for great support for exporting var)/1(x_est) -> States_estimate/1
  Demux/2 -> Transfer Fcn2/1, Mux like func (for great support for exporting var)/2(q2)
  Demux/1 -> Transfer Fcn/1, Mux like func (for great support for exporting var)/1(q1)
  Transfer Fcn2/1 -> Mux like func (for great support for exporting var)/4(dot_q2)
  Transfer Fcn/1 -> Mux like func (for great support for exporting var)/3(dot_q1)

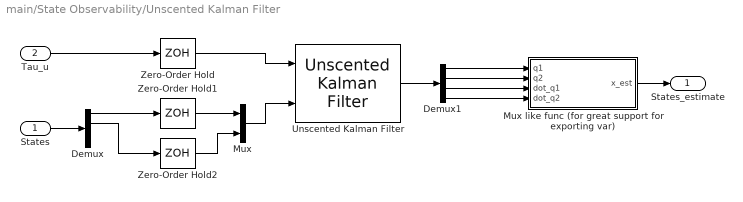
== system main/State Observability/Unscented Kalman Filter ==
  States : Inport
  Tau_u : Inport  Port=2
  Demux : Demux
  Demux1 : Demux
  Mux : Mux  Inputs=2
  Mux like func (for great support for exporting var) : MATLAB Function  TreatAsAtomicUnit=on
  Unscented Kalman Filter : sharedTrackingLibrary/Unscented Kalman Filter  StateTransitionFcn=myStateTransitionFcn  HasAdditiveProcessNoise=Additive  ProcessNoise=config.stateObservability.extKalFil.process_noise  HasTimeVaryingProcessNoise=off  HasStateTransitionFcnExtraArgument=1  InitialState=config.sim.var.init_cond.states_vec  InitialStateCovariance=config.stateObservability.extKalFil.init_state_cov  Alpha=1e-3  Beta=2  Kappa=0  MeasurementFcn1=myMeasurementFcn  HasMeasurementEnablePort1=off  HasAdditiveMeasurementNoise1=Additive  MeasurementNoise1=config.stateObservability.extKalFil.meas_noise  HasTimeVaryingMeasurementNoise1=off  HasMeasurementFcnExtraArgument1=0  HasMeasurementWrapping1=off  MeasurementFcn2=myMeasurementFcn  HasMeasurementEnablePort2=off  HasAdditiveMeasurementNoise2=Additive  MeasurementNoise2=1  HasTimeVaryingMeasurementNoise2=off  HasMeasurementFcnExtraArgument2=0  HasMeasurementWrapping2=off  MeasurementFcn3=myMeasurementFcn  HasMeasurementEnablePort3=off  HasAdditiveMeasurementNoise3=Additive  MeasurementNoise3=1  HasTimeVaryingMeasurementNoise3=off  HasMeasurementFcnExtraArgument3=0  HasMeasurementWrapping3=off  MeasurementFcn4=myMeasurementFcn  HasMeasurementEnablePort4=off  HasAdditiveMeasurementNoise4=Additive  MeasurementNoise4=1  HasTimeVaryingMeasurementNoise4=off  HasMeasurementFcnExtraArgument4=0  HasMeasurementWrapping4=off  MeasurementFcn5=myMeasurementFcn  HasMeasurementEnablePort5=off  HasAdditiveMeasurementNoise5=Additive  MeasurementNoise5=1  HasTimeVaryingMeasurementNoise5=off  HasMeasurementFcnExtraArgument5=0  HasMeasurementWrapping5=off  EnableMultirate=off  StateTransitionFcnSampleTime=1  MeasurementFcn1SampleTime=1  MeasurementFcn2SampleTime=1  MeasurementFcn3SampleTime=1  MeasurementFcn4SampleTime=1  MeasurementFcn5SampleTime=1  UseCurrentEstimator=on  OutputStateCovariance=off  DataType=double  SampleTime=config.sim.var.time_step  NumberOfMeasurements=1
      settings: LibrarySourceBlock=cstblocks/State Estimation/Unscented Kalman Filter
  Zero-Order Hold : ZeroOrderHold  SampleTime=config.sim.var.time_step
  Zero-Order Hold1 : ZeroOrderHold  SampleTime=config.sim.var.time_step
  Zero-Order Hold2 : ZeroOrderHold  SampleTime=config.sim.var.time_step
  States_estimate : Outport
  wires:
  Tau_u/1 -> Zero-Order Hold/1
  Zero-Order Hold/1 -> Unscented Kalman Filter/1
  States/1 -> Demux/1
  Demux/1 -> Zero-Order Hold1/1
  Demux/2 -> Zero-Order Hold2/1
  Mux/1 -> Unscented Kalman Filter/2
  Zero-Order Hold1/1 -> Mux/1
  Zero-Order Hold2/1 -> Mux/2
  Mux like func (for great support for exporting var)/1(x_est) -> States_estimate/1
  Unscented Kalman Filter/1 -> Demux1/1
  Demux1/1 -> Mux like func (for great support for exporting var)/1(q1)
  Demux1/2 -> Mux like func (for great support for exporting var)/2(q2)
  Demux1/3 -> Mux like func (for great support for exporting var)/3(dot_q1)
  Demux1/4 -> Mux like func (for great support for exporting var)/4(dot_q2)

== system main/External NP forces/External Disturbance Forces // Model Uncertainties/Constant Force ==
  Constant : Constant  Value=config.disturbances.external.constForce(1)
  Constant1 : Constant  Value=config.disturbances.external.constForce(2)
  Mux1 : Mux  Inputs=2
  Tau_ext : Outport
  wires:
  Constant1/1 -> Mux1/2
  Mux1/1 -> Tau_ext/1
  Constant/1 -> Mux1/1

== system main/External NP forces/External Disturbance Forces // Model Uncertainties/Gaussian Force ==
  Band-Limited White Noise (rau_2) : simulink/Sources/Band-Limited White Noise  Cov=config.disturbances.external.noise.tau_2.power  Ts=config.disturbances.external.noise.timeStep  seed=[23342]
  Band-Limited White Noise (tau_1) : simulink/Sources/Band-Limited White Noise  Cov=config.disturbances.external.noise.tau_1.power  Ts=config.disturbances.external.noise.timeStep  seed=[23341]
  Mux1 : Mux  Inputs=2
  Tau_ext : Outport
  wires:
  Band-Limited White Noise (rau_2)/1 -> Mux1/2
  Mux1/1 -> Tau_ext/1
  Band-Limited White Noise (tau_1)/1 -> Mux1/1

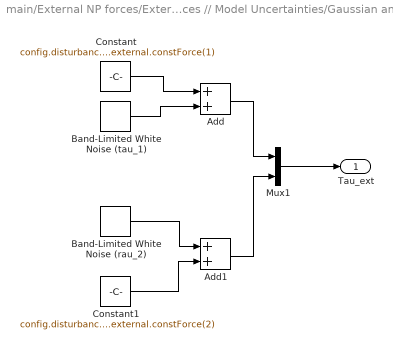
== system main/External NP forces/External Disturbance Forces // Model Uncertainties/Gaussian and Constant Force ==
  Add : Sum
  Add1 : Sum
  Band-Limited White Noise (rau_2) : simulink/Sources/Band-Limited White Noise  Cov=config.disturbances.external.noise.tau_2.power  Ts=config.disturbances.external.noise.timeStep  seed=[23342]
  Band-Limited White Noise (tau_1) : simulink/Sources/Band-Limited White Noise  Cov=config.disturbances.external.noise.tau_1.power  Ts=config.disturbances.external.noise.timeStep  seed=[23341]
  Constant : Constant  Value=config.disturbances.external.constForce(1)
  Constant1 : Constant  Value=config.disturbances.external.constForce(2)
  Mux1 : Mux  Inputs=2
  Tau_ext : Outport
  wires:
  Mux1/1 -> Tau_ext/1
  Constant/1 -> Add/1
  Band-Limited White Noise (rau_2)/1 -> Add1/1
  Constant1/1 -> Add1/2
  Add1/1 -> Mux1/2
  Band-Limited White Noise (tau_1)/1 -> Add/2
  Add/1 -> Mux1/1

== system main/External NP forces/External Disturbance Forces // Model Uncertainties/None ==
  Constant : Constant  Value=[0;0]
  Tau_ext : Outport
  wires:
  Constant/1 -> Tau_ext/1

== system main/External NP forces/Payload/None ==
  States_estimate : Inport
  Constant : Constant  Value=[0;0]
  Tau_payload : Outport
  wires:
  Constant/1 -> Tau_payload/1

== system main/External NP forces/Payload/Payload ==
  States_estimate : Inport
  Demux : Demux  Outputs=2
  Payload : MATLAB Function  TreatAsAtomicUnit=on
  Tau_payload : Outport
  wires:
  States_estimate/1 -> Demux/1
  Demux/1 -> Payload/1(q)
  Payload/1(tau_payload) -> Tau_payload/1

== matlab function main/InputSaturation/Active/Keeping the logging vector form ==
  data: tau_1 input; y output; tau_2 input
function y = fcn(tau_1, tau_2)

y = [tau_1;
     tau_2];

== matlab function main/State Observability/Unscented Kalman Filter/Mux like func (for great support for exporting var) ==
  data: q1 input; x_est output; q2 input; dot_q1 input; dot_q2 input
function x_est = fcn(q1, q2, dot_q1, dot_q2)

x_est = [q1;
         q2;
         dot_q1;
         dot_q2];

== matlab function main/Reference Generation/Trajectory/Tragectory Generation ==
  data: ref_d_TS output; t input; seg_id output; config parameter
function [ref_d_TS, seg_id] = fcn(t, config)

[ref_d_TS, seg_id] = trag_gen(t, config);

end

== matlab function main/Reference Generation/Trajectory/Switching when link "down" to "up" config. ==
  data: t input; Ref_d output; Ref_Planning input; Ref_Patch input
function Ref_d = fcn(t, Ref_Planning, Ref_Patch)
    t_init = 1.096;
    t_final = 1.572;

    if (t > t_init) && (t < t_final)
        Ref_d = Ref_Patch;
    else 
        Ref_d = Ref_Planning;
    end
end

== matlab function main/Reference Generation/Trajectory/Patch for link up//down continuity ==
  settings: updateMethod=DISCRETE  sampleTime=config.sim.var.time_step
  data: t input; Ref_Patch output; config parameter
function Ref_Patch = patch_gen(t, config)
%#codegen
% Joint-space patch between t_init and t_final using quintic interpolation.
% Output: [q1;q2;dq1;dq2;ddq1;ddq2]

t_init  = 1.096;
t_final = 1.572;
T = t_final - t_init;

% Persistent precomputation
persistent isInit c q0 dq0 ddq0 qT dqT ddqT
if isempty(isInit)
    isInit = false;
    c = zeros(2,6);
    q0 = zeros(2,1); dq0 = zeros(2,1); ddq0 = zeros(2,1);
    qT = zeros(2,1); dqT = zeros(2,1); ddqT = zeros(2,1);
end

% Precompute boundary conditions + coeffs once
if ~isInit
    % --- Boundary at t_init (DOWN) ---
    [ref0, ~] = trag_gen(t_init, config);     % ref0 = [x;y;dx;dy;ddx;ddy] :contentReference[oaicite:1]{index=1}
    p0 = ref0(1:2); v0 = ref0(3:4); a0 = ref0(5:6);

    % --- Boundary at t_final (UP) ---
    [refT, ~] = trag_gen(t_final, config);    % :contentReference[oaicite:2]{index=2}
    pT = refT(1:2); vT = refT(3:4); aT = refT(5:6);

    % Convert TS -> JS with requested elbow
    % Note: strings can be problematic for codegen in some setups.
    % If your inverse_kin uses strings and compiles, keep it.
    % Otherwise, switch to a numeric elbow flag in inverse_kin (recommended).
    [q0, dq0, ddq0] = inverse_kin(p0, v0, a0, config, "down");
    [qT, dqT, ddqT] = inverse_kin(pT, vT, aT, config, "up");

    % Unwrap final angles near initial angles to avoid 2*pi discontinuity
    qT = unwrapToRef(qT, q0);

    % Quintic coefficients for each joint
    c(1,:) = quinticCoeffs(q0(1), dq0(1), ddq0(1), qT(1), dqT(1), ddqT(1), T);
    c(2,:) = quinticCoeffs(q0(2), dq0(2), ddq0(2), qT(2), dqT(2), ddqT(2), T);

    isInit = true;
end

% Evaluate patch only over the window (outside, clamp to endpoints)
if t <= t_init
    q = q0; dq = dq0; ddq = ddq0;
elseif t >= t_final
    q = qT; dq = dqT; ddq = ddqT;
else
    tau = t - t_init;      % tau in [0,T]
    [q, dq, ddq] = evalQuintic2D(c, tau);
end

Ref_Patch = [q; dq; ddq];
end

% ===== helper functions =====

function c = quinticCoeffs(q0, dq0, ddq0, qT, dqT, ddqT, T)
% q(t)=c0+c1*t+c2*t^2+c3*t^3+c4*t^4+c5*t^5, with constraints at 0 and T
c0 = q0;
c1 = dq0;
c2 = 0.5*ddq0;

T2 = T*T; T3 = T2*T; T4 = T3*T; T5 = T4*T;

A = [   T3,    T4,    T5;
      3*T2,  4*T3,  5*T4;
      6*T,  12*T2, 20*T3];

b = [ qT  - (c0 + c1*T + c2*T2);
      dqT - (c1 + 2*c2*T);
      ddqT- (2*c2) ];

x = A \ b;
c3 = x(1); c4 = x(2); c5 = x(3);

c = [c0, c1, c2, c3, c4, c5];
end

function [q, dq, ddq] = evalQuintic2D(c, t)
q   = zeros(2,1);
dq  = zeros(2,1);
ddq = zeros(2,1);
for i = 1:2
    c0 = c(i,1); c1 = c(i,2); c2 = c(i,3);
    c3 = c(i,4); c4 = c(i,5); c5 = c(i,6);

    t2 = t*t; t3 = t2*t; t4 = t3*t; t5 = t4*t;

    q(i)   = c0 + c1*t + c2*t2 + c3*t3 + c4*t4 + c5*t5;
    dq(i)  = c1 + 2*c2*t + 3*c3*t2 + 4*c4*t3 + 5*c5*t4;
    ddq(i) = 2*c2 + 6*c3*t + 12*c4*t2 + 20*c5*t3;
end
end

function q2 = unwrapToRef(q, qref)
q2 = q;
for i = 1:2
    e = q2(i) - qref(i);
    e = mod(e + pi, 2*pi) - pi;   % wrapped error
    q2(i) = qref(i) + e;
end
end

== matlab function main/2-Link SCARA Dynamics/C(q,dot_q)dot_q/C(q,dot_q)dot_q ==
  data: q input; q_dot input; output output; config parameter
function output = fcn(q, q_dot, config)

output = c_vec(q, q_dot, config);

== matlab function main/External NP forces/Payload/Payload/Payload ==
  data: q input; tau_payload output; config parameter
function tau_payload = fcn(q, config)

    tau_payload = J_T(q, config)*W_ext(config);

end

== matlab function main/2-Link SCARA Dynamics/M^-1(q)/M^-1(q) ==
  data: q input; tau_minus_C_g_D input; output output; config parameter
function output = fcn(q, tau_minus_C_g_D, config)
    
    M_matrix = M(q, config);
    
    output = M_matrix\tau_minus_C_g_D;

== matlab function main/2-Link SCARA Dynamics/g(q)/g(q) ==
  data: q input; output output; config parameter
function output = fcn(q, config)

output = G_vec(q, config);

== matlab function main/2-Link SCARA Dynamics/D(q)/Dq_dot ==
  data: q_dot input; output output; config parameter
function output = fcn(q_dot, config)

output = D_mat(config)*q_dot;

== matlab function main/Reference Generation/Trajectory/Inverse Kinematics ==
  settings: updateMethod=DISCRETE  sampleTime=config.sim.var.time_step
  data: Ref_d_TS input; seg_id input; Ref_d_JS output; config parameter
function Ref_d_JS = fcn(Ref_d_TS, seg_id, config)
% Ref_d_TS = [x;y;dx;dy;ddx;ddy]
% Ref_d_JS = [q1;q2;dq1;dq2;ddq1;ddq2]

p = Ref_d_TS(1:2);
v = Ref_d_TS(3:4);
a = Ref_d_TS(5:6);

% Elbow switching rule:
% Up until reaching waypoint 2 (P2), then down for the last segments (P2->P4).
if seg_id <= 3
    elbow = "down";
else
    elbow = "up";
end

[q, dq, ddq] = inverse_kin(p, v, a, config, elbow);

Ref_d_JS = [q; dq; ddq];
end
